simulink model "atti"  (R2022b)
settings: Solver=FixedStepAuto  StartTime=0.0  StopTime=T  RelTol=1e-3
undefined symbols (not defined in the file or in its folder): dt, J, K, M_proc, R_mea, w_mea
libraries: shared6dof x1, aerolibutil x1
settings Model: Creator=zzy  LastModifiedBy=MoC
settings DataIOCC: ReturnWorkspaceOutputs=off

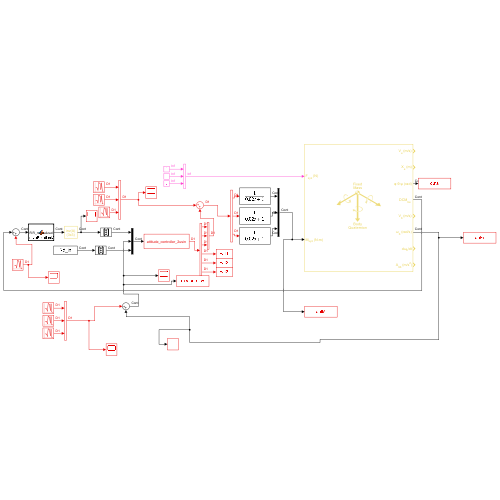
[thumbnail: Simulink's stored preview of the top-level diagram]
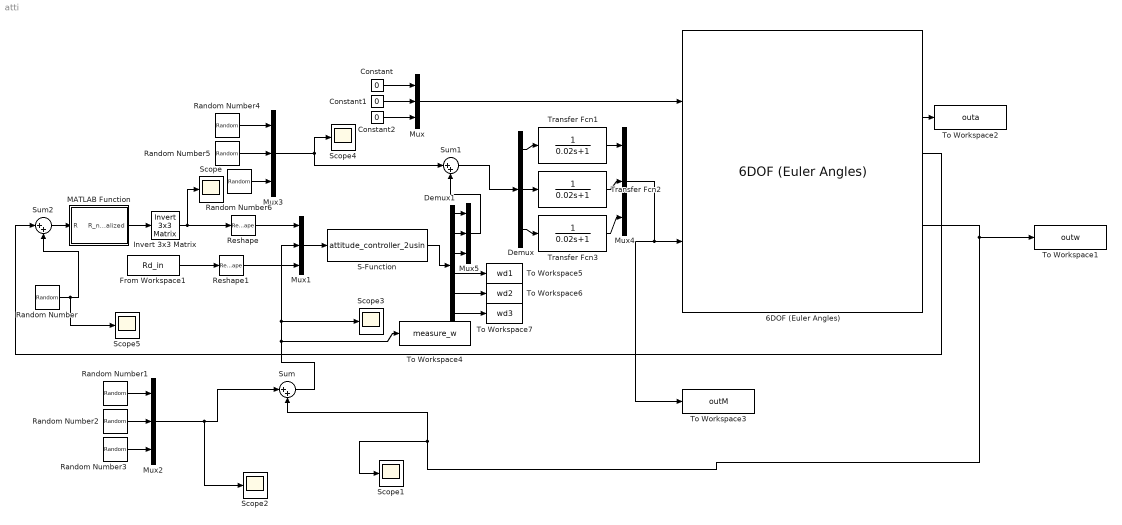
== system atti ==
  6DOF (Euler Angles) : shared6dof/6DOF (Euler Angles)  units=Metric (MKS)  mtype=Fixed  rep=Quaternion  xme_0=[0 0 0]  Vm_0=[0 0 0]  eul_0=[0 0 0]  pm_0=[0 0 0]  mass_0=1  mass_e=0.5  mass_f=2.0  inertia=J  inertia_e=eye(3)  inertia_f=2*eye(3)  k_quat=1.0  vre_flag=on  abi_flag=off  aMode=0  xme_statename=''  Vm_statename=''  eul_statename=''  quat_statename=''  pm_statename=''  mass_statename=''
  Constant : Constant  Value=0
  Constant1 : Constant  Value=0
  Constant2 : Constant  Value=0
  Demux : Demux  Outputs=3
  Demux1 : Demux  Outputs=6
  From Workspace1 : FromWorkspace  VariableName=Rd_in
  Invert 3x3 Matrix : aerolibutil/Invert  3x3 Matrix
  MATLAB Function : MATLAB Function  TreatAsAtomicUnit=on
  Mux{,1..5} (6 alike) : Mux  Inputs=3
  Random Number : RandomNumber  Variance=R_mea  SampleTime=dt
  Random Number1 : RandomNumber  Variance=w_mea  SampleTime=dt
  Random Number2 : RandomNumber  Variance=w_mea  Seed=78237  SampleTime=dt
  Random Number3 : RandomNumber  Variance=w_mea  Seed=456  SampleTime=dt
  Random Number4 : RandomNumber  Variance=M_proc  Seed=786753  SampleTime=dt
  Random Number5 : RandomNumber  Variance=M_proc  Seed=788796  SampleTime=dt
  Random Number6 : RandomNumber  Variance=M_proc  Seed=489745  SampleTime=dt
  Reshape : Reshape  OutputDimensionality=Column vector (2-D)
  Reshape1 : Reshape  OutputDimensionality=Column vector (2-D)
  S-Function : S-Function  FunctionName=attitude_controller_2usin  Parameters=dt,J,K  SFunctionDeploymentMode=off  EnableBusSupport=off
  Scope{,1..5} (6 alike) : Scope
  Sum : Sum  Inputs=|++
  Sum1 : Sum  Inputs=|++
  Sum2 : Sum  Inputs=|++
  To Workspace1 : ToWorkspace  VariableName=outw  SampleTime=-1
      settings: Save2DSignal=2-D array (concatenate along first dimension)
  To Workspace2 : ToWorkspace  VariableName=outa  SampleTime=-1
      settings: Save2DSignal=2-D array (concatenate along first dimension)
  To Workspace3 : ToWorkspace  VariableName=outM  SampleTime=-1
      settings: Save2DSignal=2-D array (concatenate along first dimension)
  To Workspace4 : ToWorkspace  VariableName=measure_w  SampleTime=-1
      settings: Save2DSignal=2-D array (concatenate along first dimension)
  To Workspace5 : ToWorkspace  VariableName=wd1  SampleTime=-1
      settings: Save2DSignal=2-D array (concatenate along first dimension)
  To Workspace6 : ToWorkspace  VariableName=wd2  SampleTime=-1
      settings: Save2DSignal=2-D array (concatenate along first dimension)
  To Workspace7 : ToWorkspace  VariableName=wd3  SampleTime=-1
      settings: Save2DSignal=2-D array (concatenate along first dimension)
  Transfer Fcn1 : TransferFcn  Denominator=[0.02 1]
  Transfer Fcn2 : TransferFcn  Denominator=[0.02 1]
  Transfer Fcn3 : TransferFcn  Denominator=[0.02 1]
  wires:
  Constant1/1 -> Mux/2
  Constant/1 -> Mux/1
  Constant2/1 -> Mux/3
  Mux/1 -> 6DOF (Euler Angles)/1
  6DOF (Euler Angles)/6 -> Sum/2, Scope1/1, To Workspace1/1
  Invert 3x3 Matrix/1 -> Scope/1, Reshape/1
  Mux1/1 -> S-Function/1
  Reshape/1 -> Mux1/1
  6DOF (Euler Angles)/3 -> To Workspace2/1
  Sum/1 -> Mux1/2, Scope3/1, To Workspace4/1
  Random Number1/1 -> Mux2/1
  Random Number2/1 -> Mux2/2
  Random Number3/1 -> Mux2/3
  Mux2/1 -> Scope2/1, Sum/1
  Random Number5/1 -> Mux3/2
  Random Number6/1 -> Mux3/3
  Random Number4/1 -> Mux3/1
  Mux3/1 -> Scope4/1, Sum1/1
  Sum1/1 -> Demux/1
  Mux4/1 -> To Workspace3/1, 6DOF (Euler Angles)/2
  Transfer Fcn2/1 -> Mux4/2
  Transfer Fcn1/1 -> Mux4/1
  Transfer Fcn3/1 -> Mux4/3
  Demux/3 -> Transfer Fcn3/1
  Demux/2 -> Transfer Fcn2/1
  Demux/1 -> Transfer Fcn1/1
  Random Number/1 -> Scope5/1, Sum2/2
  6DOF (Euler Angles)/4 -> Sum2/1
  Sum2/1 -> MATLAB Function/1(R)
  MATLAB Function/1(R_normalized) -> Invert 3x3 Matrix/1
  From Workspace1/1 -> Reshape1/1
  Reshape1/1 -> Mux1/3
  S-Function/1 -> Demux1/1
  Demux1/1 -> Mux5/1
  Demux1/2 -> Mux5/2
  Demux1/3 -> Mux5/3
  Mux5/1 -> Sum1/2
  Demux1/4 -> To Workspace5/1
  Demux1/5 -> To Workspace6/1
  Demux1/6 -> To Workspace7/1

== matlab function atti/MATLAB Function ==
  data: R input; R_normalized output
function R_normalized = normalizeRotationMatrix(R)
% Normalize a rotation matrix using SVD
    [U, ~, V] = svd(R);
    R_normalized = U * V';
end
